simulink model "ofdm_agc_mimo"  (Simulink 7.7)
settings: Solver=VariableStepDiscrete  SolverMode=SingleTasking  StartTime=0.0  StopTime=400  RelTol=1e-3
InitFcn:
  | ofdm_agc_init
StartFcn:
  | ofdm_agc_init
values from neighbouring files (symbols this model uses):
  ltbl = ltbl(2:2049)    [ofdm_agc_init.m]
undefined symbols (not defined in the file or in its folder): gcbh, xlBlockLoadCallback, xlGetNormalizedPeriod
libraries: xbsIndex_r4 x570
(part 2 of 6)

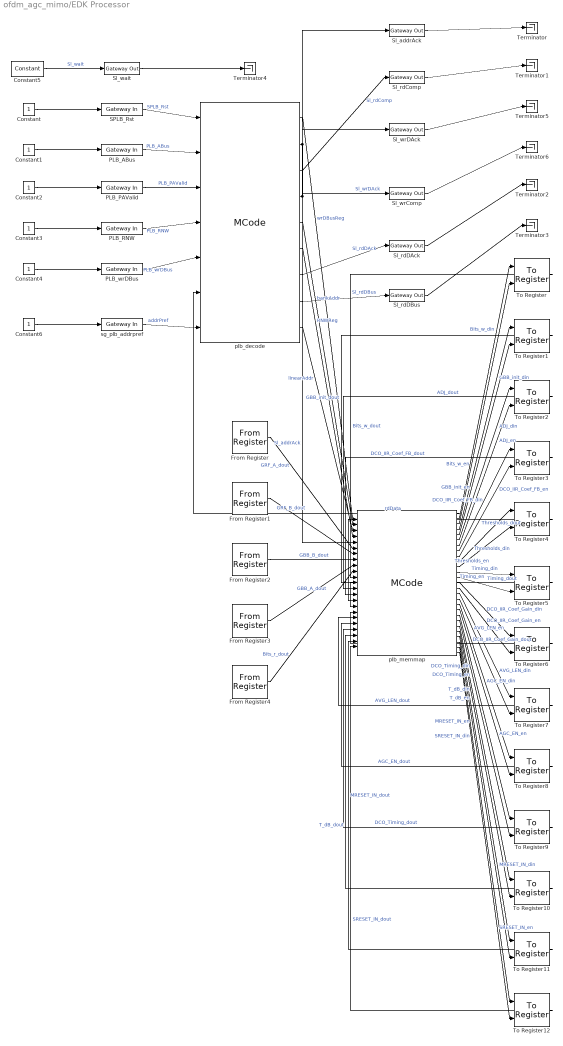
== system ofdm_agc_mimo/EDK Processor ==
  Constant{,1..4,6} (6 alike) : Constant
  Constant5 : xbsIndex_r4/Constant  const=0  gui_display_data_type=Fixed-point  arith_type=Unsigned  n_bits=1  bin_pt=0  preci_type=Single  exp_width=8  frac_width=24  explicit_period=on  period=xlGetNormalizedPeriod()  equ=P=C  opselect=C  inp2=PCIN>>17  opr=+  inp1=P  carry=CIN  dbl_ovrd=off  block_type=constant
  From Register : xbsIndex_r4/From Register  shared_memory_name='GRF_A'  init=0  period=xlGetNormalizedPeriod()  ownership=Owned and initialized elsewhere  gui_display_data_type=Fixed-point  arith_type=Unsigned  n_bits=2  bin_pt=0  preci_type=Single  dbl_ovrd=off  block_type=fromreg
      settings: AttributesFormatString=<< %<shared_memory_name> >>  infoedit="Register block that reads data to a shared memory register.  Delay of one sample period."
  From Register1 : xbsIndex_r4/From Register  shared_memory_name='GRF_B'  init=0  period=xlGetNormalizedPeriod()  ownership=Owned and initialized elsewhere  gui_display_data_type=Fixed-point  arith_type=Unsigned  n_bits=2  bin_pt=0  preci_type=Single  dbl_ovrd=off  block_type=fromreg
      settings: AttributesFormatString=<< %<shared_memory_name> >>  infoedit="Register block that reads data to a shared memory register.  Delay of one sample period."
  From Register2 : xbsIndex_r4/From Register  shared_memory_name='GBB_B'  init=0  period=xlGetNormalizedPeriod()  ownership=Owned and initialized elsewhere  gui_display_data_type=Fixed-point  arith_type=Unsigned  n_bits=5  bin_pt=0  preci_type=Single  dbl_ovrd=off  block_type=fromreg
      settings: AttributesFormatString=<< %<shared_memory_name> >>  infoedit="Register block that reads data to a shared memory register.  Delay of one sample period."
  From Register3 : xbsIndex_r4/From Register  shared_memory_name='GBB_A'  init=0  period=xlGetNormalizedPeriod()  ownership=Owned and initialized elsewhere  gui_display_data_type=Fixed-point  arith_type=Unsigned  n_bits=5  bin_pt=0  preci_type=Single  dbl_ovrd=off  block_type=fromreg
      settings: AttributesFormatString=<< %<shared_memory_name> >>  infoedit="Register block that reads data to a shared memory register.  Delay of one sample period."
  From Register4 : xbsIndex_r4/From Register  shared_memory_name='Bits_r'  init=0  period=xlGetNormalizedPeriod()  ownership=Owned and initialized elsewhere  gui_display_data_type=Fixed-point  arith_type=Unsigned  n_bits=10  bin_pt=0  preci_type=Single  dbl_ovrd=off  block_type=fromreg
      settings: AttributesFormatString=<< %<shared_memory_name> >>  infoedit="Register block that reads data to a shared memory register.  Delay of one sample period."
  PLB_ABus : xbsIndex_r4/Gateway In  gui_display_data_type=Fixed-point  arith_type=Unsigned  n_bits=32  bin_pt=0  preci_type=Single  exp_width=8  frac_width=24  quantization="Round  (unbiased: +/- Inf)"  overflow=Saturate  period=xlGetNormalizedPeriod()  dbl_ovrd=off  timing_constraint=None  locs_specified=off  LOCs={}  inherit_from_input=off  UseAsADC=off  ADCChannel='1'  hdl_port=on  block_type=gatewayin
      settings: infoedit="Gateway in block.  Converts inputs of type Simulink integer, single, double and fixed point to  Xilinx fixed-point or floating-point data type.<br><br>Hardware notes:  In hardware these blocks become top level input ports."  sginterface={'Xilinx'=>{'jtaghwcosim'=>{'non_memory_mapped_port'=>'PLB_ABus'}},'iopad'=>{'constraint'=>'#'}}
  PLB_PAValid : xbsIndex_r4/Gateway In  gui_display_data_type=Fixed-point  arith_type=Unsigned  n_bits=1  bin_pt=0  preci_type=Single  exp_width=8  frac_width=24  quantization="Round  (unbiased: +/- Inf)"  overflow=Saturate  period=xlGetNormalizedPeriod()  dbl_ovrd=off  timing_constraint=None  locs_specified=off  LOCs={}  inherit_from_input=off  UseAsADC=off  ADCChannel='1'  hdl_port=on  block_type=gatewayin
      settings: infoedit="Gateway in block.  Converts inputs of type Simulink integer, single, double and fixed point to  Xilinx fixed-point or floating-point data type.<br><br>Hardware notes:  In hardware these blocks become top level input ports."  sginterface={'Xilinx'=>{'jtaghwcosim'=>{'non_memory_mapped_port'=>'PLB_PAValid'}},'iopad'=>{'constraint'=>'#'}}
  PLB_RNW : xbsIndex_r4/Gateway In  gui_display_data_type=Fixed-point  arith_type=Unsigned  n_bits=1  bin_pt=0  preci_type=Single  exp_width=8  frac_width=24  quantization="Round  (unbiased: +/- Inf)"  overflow=Saturate  period=xlGetNormalizedPeriod()  dbl_ovrd=off  timing_constraint=None  locs_specified=off  LOCs={}  inherit_from_input=off  UseAsADC=off  ADCChannel='1'  hdl_port=on  block_type=gatewayin
      settings: infoedit="Gateway in block.  Converts inputs of type Simulink integer, single, double and fixed point to  Xilinx fixed-point or floating-point data type.<br><br>Hardware notes:  In hardware these blocks become top level input ports."  sginterface={'Xilinx'=>{'jtaghwcosim'=>{'non_memory_mapped_port'=>'PLB_RNW'}},'iopad'=>{'constraint'=>'#'}}
  PLB_wrDBus : xbsIndex_r4/Gateway In  gui_display_data_type=Fixed-point  arith_type=Unsigned  n_bits=32  bin_pt=0  preci_type=Single  exp_width=8  frac_width=24  quantization="Round  (unbiased: +/- Inf)"  overflow=Saturate  period=xlGetNormalizedPeriod()  dbl_ovrd=off  timing_constraint=None  locs_specified=off  LOCs={}  inherit_from_input=off  UseAsADC=off  ADCChannel='1'  hdl_port=on  block_type=gatewayin
      settings: infoedit="Gateway in block.  Converts inputs of type Simulink integer, single, double and fixed point to  Xilinx fixed-point or floating-point data type.<br><br>Hardware notes:  In hardware these blocks become top level input ports."  sginterface={'Xilinx'=>{'jtaghwcosim'=>{'non_memory_mapped_port'=>'PLB_wrDBus'}},'iopad'=>{'constraint'=>'#'}}
  SPLB_Rst : xbsIndex_r4/Gateway In  gui_display_data_type=Fixed-point  arith_type=Unsigned  n_bits=1  bin_pt=0  preci_type=Single  exp_width=8  frac_width=24  quantization="Round  (unbiased: +/- Inf)"  overflow=Saturate  period=xlGetNormalizedPeriod()  dbl_ovrd=off  timing_constraint=None  locs_specified=off  LOCs={}  inherit_from_input=off  UseAsADC=off  ADCChannel='1'  hdl_port=on  block_type=gatewayin
      settings: infoedit="Gateway in block.  Converts inputs of type Simulink integer, single, double and fixed point to  Xilinx fixed-point or floating-point data type.<br><br>Hardware notes:  In hardware these blocks become top level input ports."  sginterface={'Xilinx'=>{'jtaghwcosim'=>{'non_memory_mapped_port'=>'SPLB_Rst'}},'iopad'=>{'constraint'=>'#'}}
  Sl_addrAck : xbsIndex_r4/Gateway Out  inherit_from_input=off  hdl_port=on  timing_constraint=None  locs_specified=off  LOCs={}  UseAsDAC=off  DACChannel='1'  block_type=gatewayout
      settings: infoedit="Gateway out block.  Converts Xilinx fixed-point or floating-point type inputs into ouputs of type Simulink integer, single, double, or fixed point.<br><br>Hardware notes:  In hardware these blocks become top level output ports or are discarded, depending on how they are configured."  sginterface={'Xilinx'=>{'jtaghwcosim'=>{'non_memory_mapped_port'=>'Sl_addrAck'}},'iopad'=>{'constraint'=>'#'}}
  Sl_rdComp : xbsIndex_r4/Gateway Out  inherit_from_input=off  hdl_port=on  timing_constraint=None  locs_specified=off  LOCs={}  UseAsDAC=off  DACChannel='1'  block_type=gatewayout
      settings: infoedit="Gateway out block.  Converts Xilinx fixed-point or floating-point type inputs into ouputs of type Simulink integer, single, double, or fixed point.<br><br>Hardware notes:  In hardware these blocks become top level output ports or are discarded, depending on how they are configured."  sginterface={'Xilinx'=>{'jtaghwcosim'=>{'non_memory_mapped_port'=>'Sl_rdComp'}},'iopad'=>{'constraint'=>'#'}}
  Sl_rdDAck : xbsIndex_r4/Gateway Out  inherit_from_input=off  hdl_port=on  timing_constraint=None  locs_specified=off  LOCs={}  UseAsDAC=off  DACChannel='1'  block_type=gatewayout
      settings: infoedit="Gateway out block.  Converts Xilinx fixed-point or floating-point type inputs into ouputs of type Simulink integer, single, double, or fixed point.<br><br>Hardware notes:  In hardware these blocks become top level output ports or are discarded, depending on how they are configured."  sginterface={'Xilinx'=>{'jtaghwcosim'=>{'non_memory_mapped_port'=>'Sl_rdDAck'}},'iopad'=>{'constraint'=>'#'}}
  Sl_rdDBus : xbsIndex_r4/Gateway Out  inherit_from_input=off  hdl_port=on  timing_constraint=None  locs_specified=off  LOCs={}  UseAsDAC=off  DACChannel='1'  block_type=gatewayout
      settings: infoedit="Gateway out block.  Converts Xilinx fixed-point or floating-point type inputs into ouputs of type Simulink integer, single, double, or fixed point.<br><br>Hardware notes:  In hardware these blocks become top level output ports or are discarded, depending on how they are configured."  sginterface={'Xilinx'=>{'jtaghwcosim'=>{'non_memory_mapped_port'=>'Sl_rdDBus'}},'iopad'=>{'constraint'=>'#'}}
  Sl_wait : xbsIndex_r4/Gateway Out  inherit_from_input=off  hdl_port=on  timing_constraint=None  locs_specified=off  LOCs={}  UseAsDAC=off  DACChannel='1'  block_type=gatewayout
      settings: infoedit="Gateway out block.  Converts Xilinx fixed-point or floating-point type inputs into ouputs of type Simulink integer, single, double, or fixed point.<br><br>Hardware notes:  In hardware these blocks become top level output ports or are discarded, depending on how they are configured."  sginterface={'Xilinx'=>{'jtaghwcosim'=>{'non_memory_mapped_port'=>'Sl_wait'}},'iopad'=>{'constraint'=>'#'}}
  Sl_wrComp : xbsIndex_r4/Gateway Out  inherit_from_input=off  hdl_port=on  timing_constraint=None  locs_specified=off  LOCs={}  UseAsDAC=off  DACChannel='1'  block_type=gatewayout
      settings: infoedit="Gateway out block.  Converts Xilinx fixed-point or floating-point type inputs into ouputs of type Simulink integer, single, double, or fixed point.<br><br>Hardware notes:  In hardware these blocks become top level output ports or are discarded, depending on how they are configured."  sginterface={'Xilinx'=>{'jtaghwcosim'=>{'non_memory_mapped_port'=>'Sl_wrComp'}},'iopad'=>{'constraint'=>'#'}}
  Sl_wrDAck : xbsIndex_r4/Gateway Out  inherit_from_input=off  hdl_port=on  timing_constraint=None  locs_specified=off  LOCs={}  UseAsDAC=off  DACChannel='1'  block_type=gatewayout
      settings: infoedit="Gateway out block.  Converts Xilinx fixed-point or floating-point type inputs into ouputs of type Simulink integer, single, double, or fixed point.<br><br>Hardware notes:  In hardware these blocks become top level output ports or are discarded, depending on how they are configured."  sginterface={'Xilinx'=>{'jtaghwcosim'=>{'non_memory_mapped_port'=>'Sl_wrDAck'}},'iopad'=>{'constraint'=>'#'}}
  Terminator{,1..6} (7 alike) : Terminator
  To Register : xbsIndex_r4/To Register  shared_memory_name='Bits_w'  init=0  ownership=Owned and initialized elsewhere  explicit_data_type=on  gui_display_data_type=Fixed-point  arith_type=Unsigned  n_bits=10  bin_pt=0  preci_type=Single  dbl_ovrd=off  block_type=toreg
      settings: AttributesFormatString=<< %<shared_memory_name> >>  infoedit="Register block that writes data to a shared memory register.  Delay of one sample period."
  To Register1 : xbsIndex_r4/To Register  shared_memory_name='GBB_init'  init=0  ownership=Owned and initialized elsewhere  explicit_data_type=on  gui_display_data_type=Fixed-point  arith_type=Unsigned  n_bits=16  bin_pt=0  preci_type=Single  dbl_ovrd=off  block_type=toreg
      settings: AttributesFormatString=<< %<shared_memory_name> >>  infoedit="Register block that writes data to a shared memory register.  Delay of one sample period."
  To Register10 : xbsIndex_r4/To Register  shared_memory_name='T_dB'  init=0  ownership=Owned and initialized elsewhere  explicit_data_type=on  gui_display_data_type=Fixed-point  arith_type=Unsigned  n_bits=16  bin_pt=0  preci_type=Single  dbl_ovrd=off  block_type=toreg
      settings: AttributesFormatString=<< %<shared_memory_name> >>  infoedit="Register block that writes data to a shared memory register.  Delay of one sample period."
  To Register11 : xbsIndex_r4/To Register  shared_memory_name='MRESET_IN'  init=0  ownership=Owned and initialized elsewhere  explicit_data_type=on  gui_display_data_type=Fixed-point  arith_type=Unsigned  n_bits=1  bin_pt=0  preci_type=Single  dbl_ovrd=off  block_type=toreg
      settings: AttributesFormatString=<< %<shared_memory_name> >>  infoedit="Register block that writes data to a shared memory register.  Delay of one sample period."
  To Register12 : xbsIndex_r4/To Register  shared_memory_name='SRESET_IN'  init=0  ownership=Owned and initialized elsewhere  explicit_data_type=on  gui_display_data_type=Fixed-point  arith_type=Unsigned  n_bits=1  bin_pt=0  preci_type=Single  dbl_ovrd=off  block_type=toreg
      settings: AttributesFormatString=<< %<shared_memory_name> >>  infoedit="Register block that writes data to a shared memory register.  Delay of one sample period."
  To Register2 : xbsIndex_r4/To Register  shared_memory_name='ADJ'  init=0  ownership=Owned and initialized elsewhere  explicit_data_type=on  gui_display_data_type=Fixed-point  arith_type=Unsigned  n_bits=16  bin_pt=0  preci_type=Single  dbl_ovrd=off  block_type=toreg
      settings: AttributesFormatString=<< %<shared_memory_name> >>  infoedit="Register block that writes data to a shared memory register.  Delay of one sample period."
  To Register3 : xbsIndex_r4/To Register  shared_memory_name='DCO_IIR_Coef_FB'  init=0  ownership=Owned and initialized elsewhere  explicit_data_type=on  gui_display_data_type=Fixed-point  arith_type="Signed  (2's comp)"  n_bits=18  bin_pt=17  preci_type=Single  dbl_ovrd=off  block_type=toreg
      settings: AttributesFormatString=<< %<shared_memory_name> >>  infoedit="Register block that writes data to a shared memory register.  Delay of one sample period."
  To Register4 : xbsIndex_r4/To Register  shared_memory_name='Thresholds'  init=0  ownership=Owned and initialized elsewhere  explicit_data_type=on  gui_display_data_type=Fixed-point  arith_type=Unsigned  n_bits=32  bin_pt=0  preci_type=Single  dbl_ovrd=off  block_type=toreg
      settings: AttributesFormatString=<< %<shared_memory_name> >>  infoedit="Register block that writes data to a shared memory register.  Delay of one sample period."
  To Register5 : xbsIndex_r4/To Register  shared_memory_name='Timing'  init=0  ownership=Owned and initialized elsewhere  explicit_data_type=on  gui_display_data_type=Fixed-point  arith_type=Unsigned  n_bits=32  bin_pt=0  preci_type=Single  dbl_ovrd=off  block_type=toreg
      settings: AttributesFormatString=<< %<shared_memory_name> >>  infoedit="Register block that writes data to a shared memory register.  Delay of one sample period."
  To Register6 : xbsIndex_r4/To Register  shared_memory_name='DCO_IIR_Coef_Gain'  init=0  ownership=Owned and initialized elsewhere  explicit_data_type=on  gui_display_data_type=Fixed-point  arith_type=Unsigned  n_bits=18  bin_pt=17  preci_type=Single  dbl_ovrd=off  block_type=toreg
      settings: AttributesFormatString=<< %<shared_memory_name> >>  infoedit="Register block that writes data to a shared memory register.  Delay of one sample period."
  To Register7 : xbsIndex_r4/To Register  shared_memory_name='AVG_LEN'  init=0  ownership=Owned and initialized elsewhere  explicit_data_type=on  gui_display_data_type=Fixed-point  arith_type=Unsigned  n_bits=16  bin_pt=0  preci_type=Single  dbl_ovrd=off  block_type=toreg
      settings: AttributesFormatString=<< %<shared_memory_name> >>  infoedit="Register block that writes data to a shared memory register.  Delay of one sample period."
  To Register8 : xbsIndex_r4/To Register  shared_memory_name='AGC_EN'  init=0  ownership=Owned and initialized elsewhere  explicit_data_type=on  gui_display_data_type=Fixed-point  arith_type=Unsigned  n_bits=1  bin_pt=0  preci_type=Single  dbl_ovrd=off  block_type=toreg
      settings: AttributesFormatString=<< %<shared_memory_name> >>  infoedit="Register block that writes data to a shared memory register.  Delay of one sample period."
  To Register9 : xbsIndex_r4/To Register  shared_memory_name='DCO_Timing'  init=0  ownership=Owned and initialized elsewhere  explicit_data_type=on  gui_display_data_type=Fixed-point  arith_type=Unsigned  n_bits=32  bin_pt=0  preci_type=Single  dbl_ovrd=off  block_type=toreg
      settings: AttributesFormatString=<< %<shared_memory_name> >>  infoedit="Register block that writes data to a shared memory register.  Delay of one sample period."
  plb_decode : xbsIndex_r4/MCode  mfname=xlmax  explicit_period=off  period=1  dbl_ovrd=off  enable_stdout=off  enable_debug=off  mfilecontent=|  suppress_output=on  defparams={}  hide_port_list={}  block_type=mcode
      | function [wrDBusReg, addrAck, rdComp, wrDAck, bankAddr, RNWReg, rdDAck, rdDBus, linearAddr] = plb_bus_decode(plbRst, plbABus, plbPAValid, plbRNW, plbWrDBus, rdData, addrPref)
      | 
      | % constant variables (TODO: should pass from outside)
      | ADDRPREF_LEN = 20;
      | BANKADDR_LEN = 2;
      | LINEARADDR_LEN = 8;
      | ABUS_LEN = 32;
      | DBUS_LEN = 32;
      | 
      | % declare and initialize persistent variables
      | % register input bus signals
      | persistent plbRstReg_, plbRstReg_ = xl_state(0, {xlBoolean});
      | persistent plbABusReg_, plbABusReg_ = xl_state(0, {xlUnsigned, ABUS_LEN, 0});
      | persistent plbPAValidReg_, plbPAValidReg_ = xl_state(0, {xlBoolean});
      | persistent plbRNWReg_, plbRNWReg_ = xl_state(0, {xlUnsigned, 1, 0});
      | persistent plbWrDBusReg_, plbWrDBusReg_ = xl_state(0, {xlUnsigned, DBUS_LEN, 0});
      | 
      | % ===== rest of the outputs =====
      | 
      | bankAddr   = xl_slice(plbABusReg_, 2+BANKADDR_LEN+LINEARADDR_LEN-1, 2+LINEARADDR_LEN);
      | linearAddr = xl_slice(plbABusReg_, 2+LINEARADDR_LEN-1, 2);
      | RNWReg = plbRNWReg_;
      | wrDBusReg = plbWrDBusReg_;
      | 
      | % ===== p_select =====
      | 
      | % register PAValid
      | persistent aValidReg, aValidReg = xl_state(0, {xlBoolean});
      | aValidReg = plbPAValidReg_;
      | 
      | % extract and register the address prefix
      | addrPref_in = xl_slice(plbABusReg_, xl_nbits(plbABusReg_)-1, xl_nbits(plbABusReg_)-ADDRPREF_LEN);
      | if addrPref_in == addrPref
      |     ps1 = true;
      | else 
      |     ps1 = false;
      | end 
      | 
      | persistent ps1Reg, ps1Reg = xl_state(0, ps1);
      | ps1Reg = ps1;
      | 
      | ps = xl_and(ps1Reg, aValidReg);
      | 
      | % ===== addrAck =====
      | 
      | % register ps
      | persistent psReg, psReg = xl_state(0, ps);
      | 
      | addrAck = xfix({xlUnsigned, 1, 0}, xl_and(xl_not(plbRstReg_), ps, xl_not(psReg)));
      | 
      | psReg = ps;
      | 
      | % ===== rdComp, rd/wr DAck =====
      |  
      | rdComp1 = xfix({xlUnsigned, 1, 0}, xl_and(addrAck, RNWReg));
      | 
      | NUM_rdCompDelay = 3;
      | persistent rdCompDelay, rdCompDelay = xl_state(zeros(1, NUM_rdCompDelay), rdComp1, NUM_rdCompDelay);
      | rdComp2 = rdCompDelay.back;
      | rdCompDelay.push_front_pop_back(rdComp1);
      | 
      | persistent rdCompReg, rdCompReg = xl_state(0, rdComp1);
      | rdComp = rdCompReg;
      | rdCompReg = rdComp2;
      | 
      | persistent rdDAckReg, rdDAckReg = xl_state(0, rdComp1);
      | rdDAck = rdDAckReg;
      | rdDAckReg = rdComp;
      | 
      | persistent wrDAckReg, wrDAckReg = xl_state(0, addrAck);
      | wrDAck = wrDAckReg;
      | wrDAckReg = xl_and(addrAck, xl_not(RNWReg));
      | 
      | % ===== rdDBus =====
      | 
      | rdSel = xl_or(rdComp2, rdComp);
      | 
      | if rdSel == 1
      |     rdDBus1 = rdData;
      | else
      |     rdDBus1 = 0;
      | end % if
      | 
      | persistent rdDBusReg, rdDBusReg = xl_state(0, rdDBus1);
      | rdDBus = rdDBusReg;
      | rdDBusReg = rdDBus1;
      | 
      | % rdDBus = xl_concat(rdDBus32, rdDBus32);
      | % rdDBus = rdDBus32;
      | 
      | % ===== update the persistent variables =====
      | 
      | plbRstReg_ = plbRst;
      | plbABusReg_ = plbABus;
      | plbPAValidReg_ = plbPAValid;
      | plbRNWReg_ = plbRNW;
      | plbWrDBusReg_ = xl_slice(plbWrDBus, DBUS_LEN-1, 0);
  plb_memmap : xbsIndex_r4/MCode  mfname=xlmax  explicit_period=off  period=1  dbl_ovrd=off  enable_stdout=off  enable_debug=off  mfilecontent=|  suppress_output=on  defparams={}  hide_port_list={}  block_type=mcode
      | function [read_bank_out, sm_Bits_w_din, sm_Bits_w_en, sm_GBB_init_din, sm_GBB_init_en, sm_ADJ_din, sm_ADJ_en, sm_DCO_IIR_Coef_FB_din, sm_DCO_IIR_Coef_FB_en, sm_Thresholds_din, sm_Thresholds_en, sm_Timing_din, sm_Timing_en, sm_DCO_IIR_Coef_Gain_din, sm_DCO_IIR_Coef_Gain_en, sm_AVG_LEN_din, sm_AVG_LEN_en, sm_AGC_EN_din, sm_AGC_EN_en, sm_DCO_Timing_din, sm_DCO_Timing_en, sm_T_dB_din, sm_T_dB_en, sm_MRESET_IN_din, sm_MRESET_IN_en, sm_SRESET_IN_din, sm_SRESET_IN_en] = plb_memmap(wrDBus, bankAddr, linearAddr, RNWReg, addrAck, sm_GRF_A, sm_GRF_B, sm_GBB_B, sm_GBB_A, sm_Bits_r, sm_Bits_w, sm_GBB_init, sm_ADJ, sm_DCO_IIR_Coef_FB, sm_Thresholds, sm_Timing, sm_DCO_IIR_Coef_Gain, sm_AVG_LEN, sm_AGC_EN, sm_DCO_Timing, sm_T_dB, sm_MRESET_IN, sm_SRESET_IN)
      | 
      | 
      | % connvert the input data to UFix_32_0 (the bus data type)
      | % 'From Register' blocks
      | % sm_GRF_A_bus = xfix({xlUnsigned, 32, 0}, 0);
      | sm_GRF_A_bus = xl_force(sm_GRF_A, xlUnsigned, 0);
      | 
      | % sm_GRF_B_bus = xfix({xlUnsigned, 32, 0}, 0);
      | sm_GRF_B_bus = xl_force(sm_GRF_B, xlUnsigned, 0);
      | 
      | % sm_GBB_B_bus = xfix({xlUnsigned, 32, 0}, 0);
      | sm_GBB_B_bus = xl_force(sm_GBB_B, xlUnsigned, 0);
      | 
      | % sm_GBB_A_bus = xfix({xlUnsigned, 32, 0}, 0);
      | sm_GBB_A_bus = xl_force(sm_GBB_A, xlUnsigned, 0);
      | 
      | % sm_Bits_r_bus = xfix({xlUnsigned, 32, 0}, 0);
      | sm_Bits_r_bus = xl_force(sm_Bits_r, xlUnsigned, 0);
      | 
      | % 'To Register' blocks
      | 
      | % sm_Bits_w_dout = xfix({xlUnsigned, 32, 0}, 0);
      | sm_Bits_w_dout = xl_force(sm_Bits_w, xlUnsigned, 0);
      | 
      | % sm_GBB_init_dout = xfix({xlUnsigned, 32, 0}, 0);
      | sm_GBB_init_dout = xl_force(sm_GBB_init, xlUnsigned, 0);
      | 
      | % sm_ADJ_dout = xfix({xlUnsigned, 32, 0}, 0);
      | sm_ADJ_dout = xl_force(sm_ADJ, xlUnsigned, 0);
      | 
      | % sm_DCO_IIR_Coef_FB_dout = xfix({xlUnsigned, 32, 0}, 0);
      | sm_DCO_IIR_Coef_FB_dout = xl_force(sm_DCO_IIR_Coef_FB, xlUnsigned, 0);
      | 
      | % sm_Thresholds_dout = xfix({xlUnsigned, 32, 0}, 0);
      | sm_Thresholds_dout = xl_force(sm_Thresholds, xlUnsigned, 0);
      | 
      | % sm_Timing_dout = xfix({xlUnsigned, 32, 0}, 0);
      | sm_Timing_dout = xl_force(sm_Timing, xlUnsigned, 0);
      | 
      | % sm_DCO_IIR_Coef_Gain_dout = xfix({xlUnsigned, 32, 0}, 0);
      | sm_DCO_IIR_Coef_Gain_dout = xl_force(sm_DCO_IIR_Coef_Gain, xlUnsigned, 0);
      | 
      | % sm_AVG_LEN_dout = xfix({xlUnsigned, 32, 0}, 0);
      | sm_AVG_LEN_dout = xl_force(sm_AVG_LEN, xlUnsigned, 0);
      | 
      | % sm_AGC_EN_dout = xfix({xlUnsigned, 32, 0}, 0);
      | sm_AGC_EN_dout = xl_force(sm_AGC_EN, xlUnsigned, 0);
      | 
      | % sm_DCO_Timing_dout = xfix({xlUnsigned, 32, 0}, 0);
      | sm_DCO_Timing_dout = xl_force(sm_DCO_Timing, xlUnsigned, 0);
      | 
      | % sm_T_dB_dout = xfix({xlUnsigned, 32, 0}, 0);
      | sm_T_dB_dout = xl_force(sm_T_dB, xlUnsigned, 0);
      | 
      | % sm_MRESET_IN_dout = xfix({xlUnsigned, 32, 0}, 0);
      | sm_MRESET_IN_dout = xl_force(sm_MRESET_IN, xlUnsigned, 0);
      | 
      | % sm_SRESET_IN_dout = xfix({xlUnsigned, 32, 0}, 0);
      | sm_SRESET_IN_dout = xl_force(sm_SRESET_IN, xlUnsigned, 0);
      | 
      | 
      | % 'From FIFO' blocks
      | % 'To FIFO' blocks
      | % 'Shared Memory' blocks
      | 
      | % 'dout' ports of 'From Register' blocks
      | 
      | % registered register mux output
      | persistent reg_bank_out_reg; reg_bank_out_reg = xl_state(0, {xlUnsigned, 32, 0});
      | reg_bank_out = reg_bank_out_reg;
      | 
      | if linearAddr == 13
      |     reg_bank_out_reg = sm_GRF_A_bus;
      | elseif linearAddr == 14
      |     reg_bank_out_reg = sm_GRF_B_bus;
      | elseif linearAddr == 15
      |     reg_bank_out_reg = sm_GBB_B_bus;
      | elseif linearAddr == 16
      |     reg_bank_out_reg = sm_GBB_A_bus;
      | elseif linearAddr == 17
      |     reg_bank_out_reg = sm_Bits_r_bus;
      | elseif linearAddr == 0
      |     reg_bank_out_reg = sm_Bits_w_dout;
      | elseif linearAddr == 1
      |     reg_bank_out_reg = sm_GBB_init_dout;
      | elseif linearAddr == 2
      |     reg_bank_out_reg = sm_ADJ_dout;
      | elseif linearAddr == 3
      |     reg_bank_out_reg = sm_DCO_IIR_Coef_FB_dout;
      | elseif linearAddr == 4
      |     reg_bank_out_reg = sm_Thresholds_dout;
      | elseif linearAddr == 5
      |     reg_bank_out_reg = sm_Timing_dout;
      | elseif linearAddr == 6
      |     reg_bank_out_reg = sm_DCO_IIR_Coef_Gain_dout;
      | elseif linearAddr == 7
      |     reg_bank_out_reg = sm_AVG_LEN_dout;
      | elseif linearAddr == 8
      |     reg_bank_out_reg = sm_AGC_EN_dout;
      | elseif linearAddr == 9
      |     reg_bank_out_reg = sm_DCO_Timing_dout;
      | elseif linearAddr == 10
      |     reg_bank_out_reg = sm_T_dB_dout;
      | elseif linearAddr == 11
      |     reg_bank_out_reg = sm_MRESET_IN_dout;
      | elseif linearAddr == 12
      |     reg_bank_out_reg = sm_SRESET_IN_dout;
      | 
      | end
      | 
      | 
      | % 'From FIFO' and 'To FIFO' blocks
      | 
      | 
      | 
      | 
      | 
      | opCode = xl_concat(addrAck, RNWReg, bankAddr, linearAddr);
      | 
      | % 'Shared Memory' blocks
      | 
      | 
      | 
      | 
      | 
      | % 'din' ports of 'Shared Memory' blocks
      | 
      | 
      | % 'we' ports of 'Shared Memory' blocks
      | 
      | 
      | % 'addr' ports of 'Shared Memory' blocks
      | 
      | 
      | % 're' ports of 'From FIFO' blocks
      | 
      | 
      | % 'en' ports of 'To Register' blocks
      | if opCode == xl_concat(xfix({xlUnsigned, 4, 0}, 10), ...
      |                        xfix({xlUnsigned, xl_nbits(linearAddr), 0}, 0))
      |     sm_Bits_w_en = true;
      | else
      |     sm_Bits_w_en = false;
      | end
      | if opCode == xl_concat(xfix({xlUnsigned, 4, 0}, 10), ...
      |                        xfix({xlUnsigned, xl_nbits(linearAddr), 0}, 1))
      |     sm_GBB_init_en = true;
      | else
      |     sm_GBB_init_en = false;
      | end
      | if opCode == xl_concat(xfix({xlUnsigned, 4, 0}, 10), ...
      |                        xfix({xlUnsigned, xl_nbits(linearAddr), 0}, 2))
      |     sm_ADJ_en = true;
      | else
      |     sm_ADJ_en = false;
      | end
      | if opCode == xl_concat(xfix({xlUnsigned, 4, 0}, 10), ...
      |                        xfix({xlUnsigned, xl_nbits(linearAddr), 0}, 3))
      |     sm_DCO_IIR_Coef_FB_en = true;
      | else
      |     sm_DCO_IIR_Coef_FB_en = false;
      | end
      | if opCode == xl_concat(xfix({xlUnsigned, 4, 0}, 10), ...
      |                        xfix({xlUnsigned, xl_nbits(linearAddr), 0}, 4))
      |     sm_Thresholds_en = true;
      | else
      |     sm_Thresholds_en = false;
      | end
      | if opCode == xl_concat(xfix({xlUnsigned, 4, 0}, 10), ...
      |                        xfix({xlUnsigned, xl_nbits(linearAddr), 0}, 5))
      |     sm_Timing_en = true;
      | else
      |     sm_Timing_en = false;
      | end
      | if opCode == xl_concat(xfix({xlUnsigned, 4, 0}, 10), ...
      |                        xfix({xlUnsigned, xl_nbits(linearAddr), 0}, 6))
      |     sm_DCO_IIR_Coef_Gain_en = true;
      | else
      |     sm_DCO_IIR_Coef_Gain_en = false;
      | end
      | if opCode == xl_concat(xfix({xlUnsigned, 4, 0}, 10), ...
      |                        xfix({xlUnsigned, xl_nbits(linearAddr), 0}, 7))
      |     sm_AVG_LEN_en = true;
      | else
      |     sm_AVG_LEN_en = false;
      | end
      | if opCode == xl_concat(xfix({xlUnsigned, 4, 0}, 10), ...
      |                        xfix({xlUnsigned, xl_nbits(linearAddr), 0}, 8))
      |     sm_AGC_EN_en = true;
      | else
      |     sm_AGC_EN_en = false;
      | end
      | if opCode == xl_concat(xfix({xlUnsigned, 4, 0}, 10), ...
      |                        xfix({xlUnsigned, xl_nbits(linearAddr), 0}, 9))
      |     sm_DCO_Timing_en = true;
      | else
      |     sm_DCO_Timing_en = false;
      | end
      | if opCode == xl_concat(xfix({xlUnsigned, 4, 0}, 10), ...
      |                        xfix({xlUnsigned, xl_nbits(linearAddr), 0}, 10))
      |     sm_T_dB_en = true;
      | else
      |     sm_T_dB_en = false;
      | end
      | if opCode == xl_concat(xfix({xlUnsigned, 4, 0}, 10), ...
      |                        xfix({xlUnsigned, xl_nbits(linearAddr), 0}, 11))
      |     sm_MRESET_IN_en = true;
      | else
      |     sm_MRESET_IN_en = false;
      | end
      | if opCode == xl_concat(xfix({xlUnsigned, 4, 0}, 10), ...
      |                        xfix({xlUnsigned, xl_nbits(linearAddr), 0}, 12))
      |     sm_SRESET_IN_en = true;
      | else
      |     sm_SRESET_IN_en = false;
      | end
      | 
      | 
      | % 'din' ports of 'To FIFO' blocks
      | 
      | 
      | % 'we' ports of 'To FIFO' blocks
      | 
      | 
      | % 'din' ports of 'To Register' blocks
      | sm_Bits_w_din = xl_force(xl_slice(wrDBus, 10 - 1, 0), ...
      |                                  xlUnsigned, ...
      |                                  0);
      | sm_GBB_init_din = xl_force(xl_slice(wrDBus, 16 - 1, 0), ...
      |                                  xlUnsigned, ...
      |                                  0);
      | sm_ADJ_din = xl_force(xl_slice(wrDBus, 16 - 1, 0), ...
      |                                  xlUnsigned, ...
      |                                  0);
      | sm_DCO_IIR_Coef_FB_din = xl_force(xl_slice(wrDBus, 18 - 1, 0), ...
      |                                  xlSigned, ...
      |                                  17);
      | sm_Thresholds_din = xl_force(xl_slice(wrDBus, 32 - 1, 0), ...
      |                                  xlUnsigned, ...
      |                                  0);
      | sm_Timing_din = xl_force(xl_slice(wrDBus, 32 - 1, 0), ...
      |                                  xlUnsigned, ...
      |                                  0);
      | sm_DCO_IIR_Coef_Gain_din = xl_force(xl_slice(wrDBus, 18 - 1, 0), ...
      |                                  xlUnsigned, ...
      |                                  17);
      | sm_AVG_LEN_din = xl_force(xl_slice(wrDBus, 16 - 1, 0), ...
      |                                  xlUnsigned, ...
      |                                  0);
      | sm_AGC_EN_din = xl_force(xl_slice(wrDBus, 1 - 1, 0), ...
      |                                  xlUnsigned, ...
      |                                  0);
      | sm_DCO_Timing_din = xl_force(xl_slice(wrDBus, 32 - 1, 0), ...
      |                                  xlUnsigned, ...
      |                                  0);
      | sm_T_dB_din = xl_force(xl_slice(wrDBus, 16 - 1, 0), ...
      |                                  xlUnsigned, ...
      |                                  0);
      | sm_MRESET_IN_din = xl_force(xl_slice(wrDBus, 1 - 1, 0), ...
      |                                  xlUnsigned, ...
      |                                  0);
      | sm_SRESET_IN_din = xl_force(xl_slice(wrDBus, 1 - 1, 0), ...
      |                                  xlUnsigned, ...
      |                                  0);
      | 
      | 
      | persistent read_bank_out_reg; read_bank_out_reg = xl_state(0, {xlUnsigned, 32, 0});
      | read_bank_out = read_bank_out_reg;
      | 
      | persistent bankAddr_reg; bankAddr_reg = xl_state(0, bankAddr);
      | 
      | if bankAddr_reg == 0
      |     % Bank 0: Shared Memories
      |     read_bank_out_reg = 0;
      | elseif bankAddr_reg == 1
      |     % Bank 1: From/To FIFOs
      |     read_bank_out_reg =  0;
      | elseif bankAddr_reg == 2
      |     % Bank 2: From/To Registers
      |     read_bank_out_reg = reg_bank_out;
      | elseif bankAddr_reg == 3
      |     % Bank 3: Configuration Registers
      |     read_bank_out_reg = 0;
      | end
      | 
      | bankAddr_reg = bankAddr;
  sg_plb_addrpref : xbsIndex_r4/Gateway In  gui_display_data_type=Fixed-point  arith_type=Unsigned  n_bits=20  bin_pt=0  preci_type=Single  exp_width=8  frac_width=24  quantization="Round  (unbiased: +/- Inf)"  overflow=Saturate  period=xlGetNormalizedPeriod()  dbl_ovrd=off  timing_constraint=None  locs_specified=off  LOCs={}  inherit_from_input=off  UseAsADC=off  ADCChannel='1'  hdl_port=on  block_type=gatewayin
      settings: infoedit="Gateway in block.  Converts inputs of type Simulink integer, single, double and fixed point to  Xilinx fixed-point or floating-point data type.<br><br>Hardware notes:  In hardware these blocks become top level input ports."  sginterface={'Xilinx'=>{'jtaghwcosim'=>{'non_memory_mapped_port'=>'sg_plb_addrpref'}},'iopad'=>{'constraint'=>'#'}}
  wires:
  plb_decode/2 -> plb_memmap/5, Sl_addrAck/1  "Sl_addrAck"
  plb_decode/4 -> Sl_wrDAck/1, Sl_wrComp/1  "Sl_wrDAck"
  plb_memmap/27 -> To Register12/2  "SRESET_IN_en"
  plb_memmap/26 -> To Register12/1  "SRESET_IN_din"
  plb_memmap/25 -> To Register11/2  "MRESET_IN_en"
  plb_memmap/24 -> To Register11/1  "MRESET_IN_din"
  plb_memmap/23 -> To Register10/2  "T_dB_en"
  plb_memmap/22 -> To Register10/1  "T_dB_din"
  plb_memmap/21 -> To Register9/2  "DCO_Timing_en"
  plb_memmap/20 -> To Register9/1  "DCO_Timing_din"
  plb_memmap/19 -> To Register8/2  "AGC_EN_en"
  plb_memmap/18 -> To Register8/1  "AGC_EN_din"
  plb_memmap/17 -> To Register7/2  "AVG_LEN_en"
  plb_memmap/16 -> To Register7/1  "AVG_LEN_din"
  plb_memmap/15 -> To Register6/2  "DCO_IIR_Coef_Gain_en"
  plb_memmap/14 -> To Register6/1  "DCO_IIR_Coef_Gain_din"
  plb_memmap/13 -> To Register5/2  "Timing_en"
  plb_memmap/12 -> To Register5/1  "Timing_din"
  plb_memmap/11 -> To Register4/2  "Thresholds_en"
  plb_memmap/10 -> To Register4/1  "Thresholds_din"
  plb_memmap/9 -> To Register3/2  "DCO_IIR_Coef_FB_en"
  plb_memmap/8 -> To Register3/1  "DCO_IIR_Coef_FB_din"
  plb_memmap/7 -> To Register2/2  "ADJ_en"
  plb_memmap/6 -> To Register2/1  "ADJ_din"
  plb_memmap/5 -> To Register1/2  "GBB_init_en"
  plb_memmap/4 -> To Register1/1  "GBB_init_din"
  plb_memmap/3 -> To Register/2  "Bits_w_en"
  plb_memmap/2 -> To Register/1  "Bits_w_din"
  plb_memmap/1 -> plb_decode/6  "rdData"
  To Register12/1 -> plb_memmap/23  "SRESET_IN_dout"
  To Register11/1 -> plb_memmap/22  "MRESET_IN_dout"
  To Register10/1 -> plb_memmap/21  "T_dB_dout"
  To Register9/1 -> plb_memmap/20  "DCO_Timing_dout"
  To Register8/1 -> plb_memmap/19  "AGC_EN_dout"
  To Register7/1 -> plb_memmap/18  "AVG_LEN_dout"
  To Register6/1 -> plb_memmap/17  "DCO_IIR_Coef_Gain_dout"
  To Register5/1 -> plb_memmap/16  "Timing_dout"
  To Register4/1 -> plb_memmap/15  "Thresholds_dout"
  To Register3/1 -> plb_memmap/14  "DCO_IIR_Coef_FB_dout"
  To Register2/1 -> plb_memmap/13  "ADJ_dout"
  To Register1/1 -> plb_memmap/12  "GBB_init_dout"
  To Register/1 -> plb_memmap/11  "Bits_w_dout"
  From Register4/1 -> plb_memmap/10  "Bits_r_dout"
  From Register3/1 -> plb_memmap/9  "GBB_A_dout"
  From Register2/1 -> plb_memmap/8  "GBB_B_dout"
  From Register1/1 -> plb_memmap/7  "GRF_B_dout"
  From Register/1 -> plb_memmap/6  "GRF_A_dout"
  plb_decode/6 -> plb_memmap/4  "RNWReg"
  plb_decode/9 -> plb_memmap/3  "linearAddr"
  plb_decode/5 -> plb_memmap/2  "bankAddr"
  plb_decode/1 -> plb_memmap/1  "wrDBusReg"
  plb_decode/8 -> Sl_rdDBus/1  "Sl_rdDBus"
  plb_decode/7 -> Sl_rdDAck/1  "Sl_rdDAck"
  plb_decode/3 -> Sl_rdComp/1  "Sl_rdComp"
  sg_plb_addrpref/1 -> plb_decode/7  "addrPref"
  PLB_wrDBus/1 -> plb_decode/5  "PLB_wrDBus"
  PLB_RNW/1 -> plb_decode/4  "PLB_RNW"
  PLB_PAValid/1 -> plb_decode/3  "PLB_PAValid"
  PLB_ABus/1 -> plb_decode/2  "PLB_ABus"
  SPLB_Rst/1 -> plb_decode/1  "SPLB_Rst"
  Constant6/1 -> sg_plb_addrpref/1
  Constant5/1 -> Sl_wait/1  "Sl_wait"
  Constant4/1 -> PLB_wrDBus/1
  Constant3/1 -> PLB_RNW/1
  Constant2/1 -> PLB_PAValid/1
  Constant1/1 -> PLB_ABus/1
  Constant/1 -> SPLB_Rst/1
  Sl_wrComp/1 -> Terminator6/1
  Sl_wrDAck/1 -> Terminator5/1
  Sl_wait/1 -> Terminator4/1
  Sl_rdDBus/1 -> Terminator3/1
  Sl_rdDAck/1 -> Terminator2/1
  Sl_rdComp/1 -> Terminator1/1
  Sl_addrAck/1 -> Terminator/1
